simulink model "synth_hinf_ctrl_lin_uncertain_model_z"  (R2020b)
settings: Solver=VariableStepAuto  StartTime=0.0  StopTime=10.0  RelTol=1e-3
values from neighbouring files (symbols this model uses):
  B = 10    [hinfCostFunc.m]    (also in hinf_analysis_z.m; hinf_cmd_lmi.m = [zeros(4,2); Sigma.B]; init_rob_synth_sim.m; muCostFunc.m = 11)
  dq0 = [0;0;0]    [hinfCostFunc.m]    (also in hinf_analysis_z.m; init_rob_synth_sim.m = [0; 0; 0]; muCostFunc.m; mu_analysis_z.m)
  M = 0.45    [hinfCostFunc.m]    (also in hinf_analysis_z.m; init_rob_synth_sim.m; muCostFunc.m = 0.42; mu_analysis_z.m = 0.42)
  q0 = [1.676; -4.363; 1.497]    [hinfCostFunc.m]    (also in hinf_analysis_z.m; init_rob_synth_sim.m; muCostFunc.m; mu_analysis_z.m)
  Sigma = minreal(Sigma, [], false)    [hinfCostFunc.m]    (also in hinf_analysis_z.m = youbot_lin_model_ss_z; hinf_cmd_lmi.m = youbot_lin_model_ss_z; muCostFunc.m; mu_analysis_z.m = youbot_lin_model_ss_z)
  tau_m = 1/(10*2*pi)    (= 0.0159154943092)    [hinfCostFunc.m]    (also in hinf_analysis_z.m; init_rob_synth_sim.m; muCostFunc.m; mu_analysis_z.m)
  W1 = 1/makeweight(1e-6,[2*pi*fc_w1,1],g_w1,0,2)    [hinfCostFunc.m]    (also in hinf_analysis_z.m = 1/makeweight(1e-6,[2*pi*x(1),1],x(3),0,2); init_rob_synth_sim.m = makeweight(1.5,[2*pi*3,1],0); muCostFunc.m; mu_analysis_z.m = 1/makeweight(1e-6,[2*pi*x(1),1],x(3),0,2))
  W2 = 1/makeweight(g_w2,[2*pi*fc_w2,1],0.1)    [hinfCostFunc.m]    (also in hinf_analysis_z.m = 1/makeweight(x(4),[2*pi*x(2),1],0.1); init_rob_synth_sim.m = makeweight(1.5,[2*pi*3,1],0); muCostFunc.m; mu_analysis_z.m = 1/makeweight(x(4),[2*pi*x(2),1],0.1))
libraries: RCTblocks x1
settings Model: Creator=Fortineau_Vin  LastModifiedBy=Fortineau_Vin

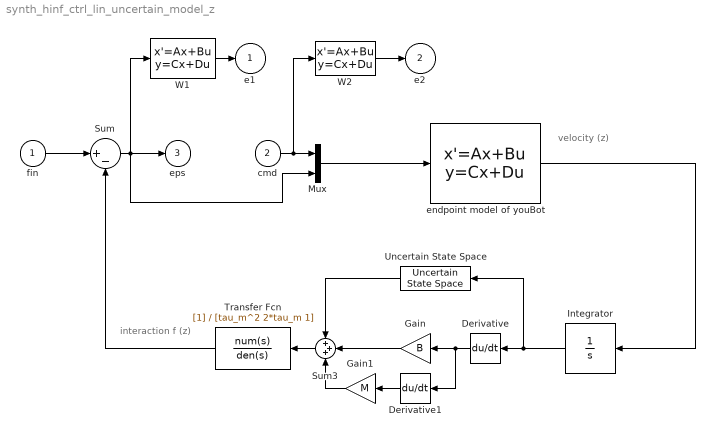
== system synth_hinf_ctrl_lin_uncertain_model_z ==
  note: velocity (z)
  note: interaction f (z)
  fin : Inport  PortDimensions=1
  cmd : Inport  Port=2  PortDimensions=1
  Derivative : Derivative
  Derivative1 : Derivative
  Gain : Gain  Gain=B
  Gain1 : Gain  Gain=M
  Integrator : Integrator
  Mux : Mux  Inputs=2
  Sum : Sum  Inputs=|+-
  Sum3 : Sum  Inputs=+++
  Transfer Fcn : TransferFcn  Denominator=[tau_m^2 2*tau_m 1]
  Uncertain State Space : RCTblocks/Uncertain State Space  Tag=USS  USystem=K  UValue=[]  X0=[]  uX0=[]
      settings: SourceProductBaseCode=RC
  W1 : StateSpace  A=W1.A  B=W1.B  C=W1.C  D=W1.D  InitialCondition=0
  W2 : StateSpace  A=W2.A  B=W2.B  C=W2.C  D=W2.D  InitialCondition=0
  endpoint model of youBot : StateSpace  A=Sigma.A  B=Sigma.B  C=Sigma.C  D=Sigma.D  InitialCondition=[q0;dq0]
  e1 : Outport  PortDimensions=1
  e2 : Outport  Port=2  PortDimensions=1
  eps : Outport  Port=3
  wires:
  endpoint model of youBot/1 -> Integrator/1
  Sum/1 -> Mux/2, eps/1, W1/1
  Mux/1 -> endpoint model of youBot/1
  W1/1 -> e1/1
  Transfer Fcn/1 -> Sum/2
  W2/1 -> e2/1
  fin/1 -> Sum/1
  cmd/1 -> W2/1, Mux/1
  Gain/1 -> Sum3/2
  Integrator/1 -> Derivative/1, Uncertain State Space/1
  Derivative/1 -> Derivative1/1, Gain/1
  Gain1/1 -> Sum3/3
  Sum3/1 -> Transfer Fcn/1
  Uncertain State Space/1 -> Sum3/1
  Derivative1/1 -> Gain1/1
